simulink model "crazy_model_controller_pid"  (R2014b)
settings: Solver=ode4  StartTime=0.0  StopTime=10  FixedStep=0.01  RelTol=1e-3
values from neighbouring files (symbols this model uses):
  Kv = 14000*[1 0 0 0 ... (first row only)    [control_PWM.m]    (also in linearize_pwm.m = 14000; linearize_voltage.m = 14000)
settings Model: Creator=Abhiram  LastModifiedBy=Abhiram

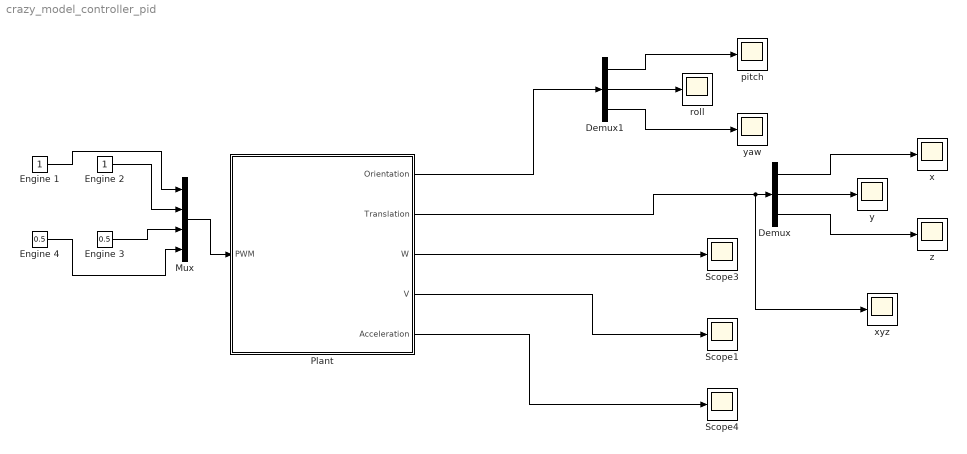
== system crazy_model_controller_pid ==
  Demux : Demux  Outputs=3
  Demux1 : Demux  Outputs=3
  Engine 1 : Constant
  Engine 2 : Constant
  Engine 3 : Constant  Value=0.5
  Engine 4 : Constant  Value=0.5
  Mux : Mux
  Plant : Subsystem
  Scope1 : Scope
  Scope3 : Scope
      settings: SaveName=ScopeData3
  Scope4 : Scope
      settings: SaveName=ScopeData4
  pitch : Scope
  roll : Scope
      settings: TimeRange=10  YMin=0  YMax=25  SaveName=ScopeData7
  x : Scope
      settings: SaveName=ScopeData2
  xyz : Scope
      settings: SaveName=ScopeData9
  y : Scope
      settings: SaveName=ScopeData5
  yaw : Scope
      settings: SaveName=ScopeData8
  z : Scope
      settings: SaveName=ScopeData6
  wires:
  Plant/1(Orientation) -> Demux1/1
  Plant/3(W) -> Scope3/1
  Plant/4(V) -> Scope1/1
  Plant/5(Acceleration) -> Scope4/1
  Plant/2(Translation) -> Demux/1, xyz/1
  Demux/1 -> x/1
  Demux/2 -> y/1
  Demux/3 -> z/1
  Demux1/1 -> pitch/1
  Demux1/2 -> roll/1
  Demux1/3 -> yaw/1
  Engine 1/1 -> Mux/1
  Engine 2/1 -> Mux/2
  Engine 3/1 -> Mux/3
  Engine 4/1 -> Mux/4
  Mux/1 -> Plant/1(PWM)

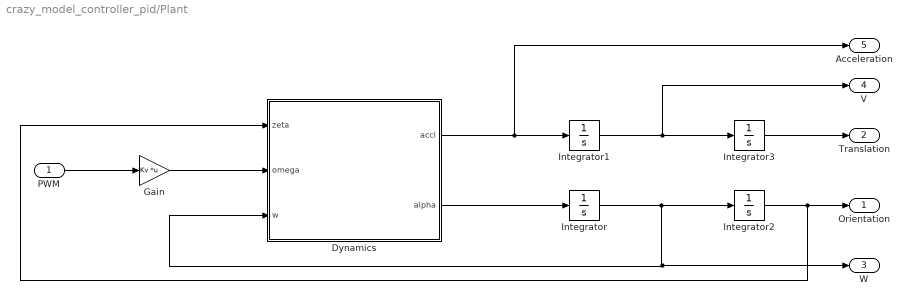
== system crazy_model_controller_pid/Plant ==
  PWM : Inport
  Dynamics : MATLAB Function  TreatAsAtomicUnit=on
  Gain : Gain  Gain=Kv  Multiplication=Matrix(K*u)
  Integrator{,1..3} (4 alike) : Integrator  InitialCondition=[0 0 0]'
  Orientation : Outport
  Translation : Outport  Port=2
  W : Outport  Port=3
  V : Outport  Port=4
  Acceleration : Outport  Port=5
  wires:
  Integrator/1 -> Integrator2/1, Dynamics/3(w), W/1
  Integrator1/1 -> V/1, Integrator3/1
  Integrator2/1 -> Dynamics/1(zeta), Orientation/1
  Integrator3/1 -> Translation/1
  PWM/1 -> Gain/1
  Dynamics/2(alpha) -> Integrator/1
  Dynamics/1(accl) -> Acceleration/1, Integrator1/1
  Gain/1 -> Dynamics/2(omega)

== matlab function crazy_model_controller_pid/Plant/Dynamics ==
  data: zeta input; omega input; accl output; alpha output; w input
function [accl, alpha] = fcn(zeta, omega, w)

    % w unknown - how to get it
    % modelling and control of mini flying machines

%     accl = [0 0 0]';
%     alpha = [0 0 0]';

    Ct = 10;
    Cq = 10;
    d = 0.05;
    m = 0.1;
    g = 9.8;
    % Inertia = ?

    C = [Ct     Ct    Ct    Ct;
         0      d*Ct  0     -d*Ct;
        -d*Ct   0     d*Ct  0;
        -Cq     Cq   -Cq    Cq ]; % Plus config

%%%%%%%%%%%%%%%%%%%%%%%%%%%%%%%%%%%%%%%%%%%    
% % % 1    
% % %     psi = zeta(1);           % yaw
% % %     phi = zeta(2);           % roll
% % %     theta = zeta(3);         % pitch
% %     
% % %2    
% % %     psi = zeta(1);           % yaw
% % %     theta = zeta(2);         % pitch
% % %     phi = zeta(3);           % roll

%3
    theta = zeta(1);         % pitch    
    phi = zeta(2);           % roll
    psi = zeta(3);           % yaw
%%%%%%%%%%%%%%%%%%%%%%%%%%%%%%%%%%%%%%%%%%%%%


% Rotation matrix 1 from the slides
% R =  [cos(psi)*cos(theta)-sin(phi)*sin(psi)*sin(theta)      -cos(phi)*sin(psi)      cos(psi)*sin(theta)+cos(theta)*sin(phi)*sin(psi);
%           cos(theta)*cos(psi)-cos(psi)*sin(phi)*sin(theta)       cos(phi)*cos(psi)      sin(psi)*sin(theta)-cos(psi)*cos(theta)*sin(phi);
%           -cos(phi)*sin(theta)                                   sin(phi)               cos(phi)*cos(theta)                            ];

% Rotation matrix 2 from the slides
% R = [ cos(psi)*cos(theta), cos(psi)*sin(phi)*sin(theta) - cos(phi)*sin(psi), sin(phi)*sin(psi) + cos(phi)*cos(psi)*sin(theta);
%       cos(theta)*sin(psi), cos(phi)*cos(psi) + sin(phi)*sin(psi)*sin(theta), cos(phi)*sin(psi)*sin(theta) - cos(psi)*sin(phi);
%      -sin(theta),                              cos(theta)*sin(phi),                              cos(phi)*cos(theta)];      

omega_square = [omega(1)^2 omega(2)^2 omega(3)^2 omega(4)^2]';
T_b = C*omega_square;

%     F_b = [0 0 T_b(1)]';
%     F_e = R*F_b;

    F_e = T_b(1)*[-sin(theta); cos(theta)*sin(phi); cos(theta)*cos(phi)];
    
    
    Tau_e = [T_b(2) T_b(3) T_b(4)]';
    G = [0 0 m*g]';

    T_e = [F_e - G; Tau_e];
    I = eye(3);                                 % Inertia matrix - needs revision

    I_a = [m*eye(3)    zeros(3,3);
           zeros(3,3)         I ];

    w_cross = cross(w,I*w);

    % Needs Revision
    A = I_a \ ( T_e - [0;0;0;w_cross] );
    
    accl = A(1:3);
    alpha = A(4:6);

end
